simulink model "GTA_PCMFirmware"  (Simulink 7.8)
settings: Solver=FixedStepDiscrete  StartTime=0.0  StopTime=10.0  RelTol=1e-3
PreLoadFcn:
  | try, eval([bdroot '_setup']); catch, eval('model_setup', ''); end
InitFcn:
  | try, eval([bdroot '_setup']); catch, eval('model_setup', ''); end
undefined symbols (not defined in the file): fndFwd, fndNeut, fndRev, FWDlockout, GCM, keySwIgn2, motohawk_build_version, motohawk_trunc_name, motohawk_vardec_path, REVlockout
libraries: MotoHawk_lib x313, simulink x47, GTA_Library x13
(part 1 of 7)
Description:
  | GTA_PCMFirmware
CloseFcn:
  | try, eval([bdroot '_close']); catch, eval('model_close', ''); end
settings Model: MotoHawkBuildVersion=020  MotoHawkBuildStats=struct('TotalFLASH',{0},'TotalEEPROM',{0},'TotalRAM',{0},'AppFLASH',{0},'AppEEPROM',{0},'AppRAM',{0},'HeapRAM',{0},'BuildSuccessCount',{20},'BuildErrorCount',{3})  MotoHawkModelSavedName=GTA_PCMFirmware  MotoHawkModelGUID=31d1e75d-84c7-4dc1-83-eb-d3-41-88-c6-07  MotoHawkModelOpenTime=2012 8 2 11 56 57.463  MotoHawkModelElapsedTime=1635613.383  MotoHawkBuildInfo=struct('model_name',{'GTA_PCMFirmware'},'motohawk_version',{'2011b_sp2.227'},'motohawk_component_version',{'0.0.7'},'matlab_version',{'7.13.0'},'build_version',{'019'},'module_type',{'GCM-0563-048-0802'},'layout_type',{'DEV'},'processor_family',{'PPC'},'processor_type',{'MPC563'},'toolchain_vendor',{'gcc-powerpc-eabi'},'toolchain_version',{'4.6.0'},'component',{0},'archive_file',{'FIRE48.a'},'enable_build',{1},'fptype',{0},'flash_size',{524288},'ee_size',{16384},'ram_size',{32768},'decram_size',{2048},'module_memory_def',{'MPC563_ModMemoryDef_Dev'},'eri_table0_rev',{9},'max_eri_table_size',{65535},'use_debug_vardecs',{1},'use_info_vardecs',{1},'fgnd_base_period_ms',{5},'bgnd_base_period_ms',{50},'root_build_dir',{'D:\Users\pipenberg\Dropbox\WMGTA\Technical\Software\PCM_Firmware\GTA_PCMFirmware'},'build_dir',{'D:\Users\pipenberg\Dropbox\WMGTA\Technical\Software\PCM_Firmware\GTA_PCMFirmware\GTA_PCMFirmware_Build'},'dll_name',{'GTA_PCMFi_019'},'srz_name',{'GTA_PCMFirmware_019'},'fgnd_stack_size',{3072},'fgnd_angle_stack_size',{0},'bgnd_stack_size',{2048},'idle_stack_size',{1024},'irq_stack_size',{1536},'heap_size',{4096},'heap_margin',{409},'install_dll_dir',{'C:\ECUFiles\TDBDLL'},'install_srz_dir',{'C:\ECUFiles\Programs\'},'app_int_stack_size',{1024},'shutdown_stack_size',{1024},'mingw_dir',{'C:\Program Files (x86)\Woodward\DevelopmentTools\Toolchains\GCC\win32-pe\4_4_0\'},'motohawk_dir',{'C:\Program Files (x86)\Woodward\MCS\MotoHawk\2011b_sp2.227'},'toolchain_dir',{'C:\Program Files (x86)\Woodward\DevelopmentTools\Toolchains\GCC\powerpc-eabi\4_6_0'},'matlab_root',{'C:\Program Files\MATLAB\R2011b'},'model_guid',{'31d1e75d-84c7-4dc1-83-eb-d3-41-88-c6-07'},'build_guid',{'afea414d-dbf6-4ed7-b0-f9-6e-db-88-3a-76'},'token_guid',{'71C461C96109B340859695742C634452'})  MotoHawkBuildGUID=afea414d-dbf6-4ed7-b0-f9-6e-db-88-3a-76  Creator=cspenc  LastModifiedBy=pipenberg
settings OptimizationCC: InlineParams=on  InitFltsAndDblsToZero=on  OptimizeModelRefInitCode=on  LifeSpan=1
settings DebuggingCC: SolverPrmCheckMsg=none  InheritedTsInSrcMsg=none  TasksWithSamePriorityMsg=none  FcnCallInpInsideContextMsg=Use local settings  StrictBusMsg=Warning
settings HardwareCC: ProdEndianess=BigEndian  ProdHWDeviceType=Specified
settings RTWCC: SystemTargetFile=motohawk_ert_rtw.tlc  TLCOptions="-aCustomNonFinites=\"motohawk_genrtnonfinite.tlc\""  MakeCommand=motohawk_make_rtw  TemplateMakefile=motohawk_ert_rtw.tmf  Description=MotoHawk(tm) Rapid Prototyping  ProcessScript=motohawk_ert_rtw_make_rtw_hook
settings CodeAppCC: IgnoreCustomStorageClasses=off  MaxIdLength=100  CustomSymbolStrField=$H$N$M
settings STFCustomTargetCC: ModelReferenceCompliant=off  GeneratePreprocessorConditionals=Use local settings  CombineOutputUpdateFcns=on  ERTCustomFileBanners=on  SupportContinuousTime=off  SupportNonInlinedSFcns=off  CPPClassGenCompliant=on  SystemTargetFile=motohawk_ert_rtw.tlc
settings ERTTargetCC: MultiwordLength=2048  ModelReferenceCompliant=off  ParMdlRefBuildCompliant=off  CompOptLevelCompliant=off  ConcurrentExecutionCompliant=off  ERTFirstTimeCompliant=off  ModelStepFunctionPrototypeControlCompliant=off  ERTCustomFileTemplate=example_file_process.tlc  ConvertIfToSwitch=off  SuppressUnreachableDefaultCases=off

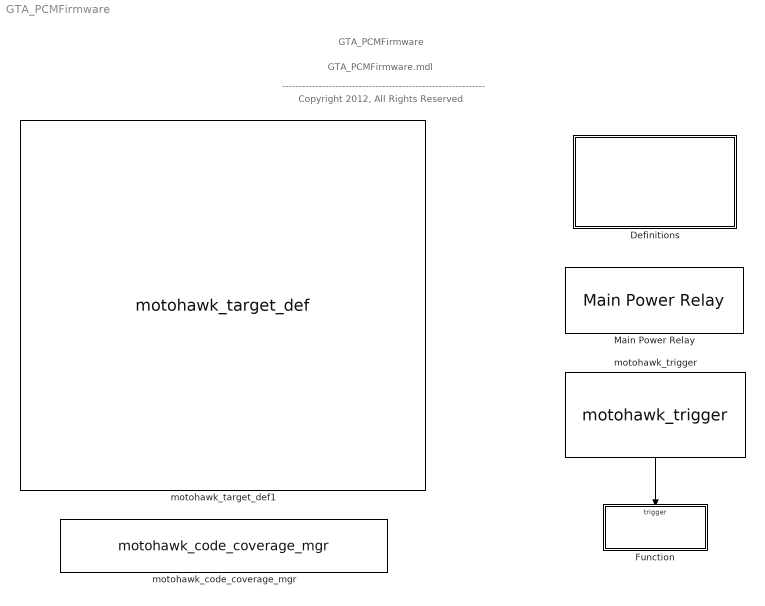
== system GTA_PCMFirmware ==
  note: GTA_PCMFirmware
  note: GTA_PCMFirmware.mdl
  note: -------------------------------------------------------------
  note: Copyright 2012, All Rights Reserved
  Definitions : Subsystem
  Function : Subsystem  TreatAsAtomicUnit=on
      mask init:
      | SampleTime = 0.005;
      | lbl = sprintf('%d ms', SampleTime * 1000);
      settings: RTWSystemCode=Function  RTWFcnNameOpts=Use subsystem name  RTWFileNameOpts=Use function name
      mask Display: disp(lbl);
  Main Power Relay : MotoHawk_lib/Extra Development Blocks/Main Power Relay  on_delay_count=2  off_delay_count=5  ecup_threshold=100  group='System | Main Power Relay'
  motohawk_code_coverage_mgr : MotoHawk_lib/Extra Development Blocks/motohawk_code_coverage_mgr  codegen=Always Generate Code Coverage Code  group='System | Code Coverage'
  motohawk_target_def1 : MotoHawk_lib/motohawk_target_def  Priority=-65535  target=GCM-0563-048-0802  layout=DEV  fptype=single (32 bits)  fgnd_stack_size=3*1024  fgnd_angle_stack_size=0  bgnd_stack_size=2*1024  idle_stack_size=1024  irq_stack_size=1536  app_int_stack_size=1024  shutdown_stack_size=1024  heap_size=4*1024  show_margins=off  fgnd_stack_margin=(3*1024) * 0.1  fgnd_angle_stack_margin=0  bgnd_stack_margin=(2*1024) * 0.1  idle_stack_margin=(1024) * 0.1  irq_stack_margin=(1536) * 0.1  app_int_stack_margin=(1024) * 0.1  shutdown_stack_margin=(1024) * 0.1  heap_margin=(4*1024) * 0.1  comp_name=bdroot  comp_img='KVASER_CAN_USB.jpg'  comp_security=No Encryption  comp_build_pass='mhbuild'  comp_sim_pass='mhsim'  comp_multi=off  show_filenames=off  dll_name=motohawk_trunc_name(bdroot, ['_' motohawk_build_version], 13)  srz_name=motohawk_trunc_name(bdroot, ['_' motohawk_build_version], 50)  build_dir='.'  comp_dir='.'
  motohawk_trigger : MotoHawk_lib/Trigger Blocks/motohawk_trigger  Tag=Trigger  Priority=0  trigger=FGND_RTI_PERIODIC  function_name=Trigger_FGND_RTI_PERIODIC_8744p0012  priority_order=0  inherited=off  run_disabled=off  override_app_monitor=off  target=GCM_0563_048_0802
  wires:
  motohawk_trigger/1 -> Function/Trigger

== system GTA_PCMFirmware/Definitions ==
  CAN Definition : MotoHawk_lib/CAN Blocks/CAN Definition  Priority=-100  nam='CAN_1'  text_resource=CAN1  code_resource=NONE  val_resource=-1  target=GCM-0563-048-0802  bus=-2  btime=500 kbaud  pre=1  prop=0  pseg1=0  pseg2=0  resyn=0  tx_queue_size=16  rx_queue_size=16  use_protocol=on  city_id=hex2dec('B')  access_level=4  mototune_group='System | System Config | Communication Config'
  CAN Definition1 : MotoHawk_lib/CAN Blocks/CAN Definition  Priority=-100  nam='BMS_CAN'  text_resource=CAN2  code_resource=NONE  val_resource=-1  target=GCM-0563-048-0802  bus=-2  btime=500 kbaud  pre=1  prop=0  pseg1=0  pseg2=0  resyn=0  tx_queue_size=16  rx_queue_size=16  use_protocol=on  city_id=hex2dec('B')  access_level=4  mototune_group='System | System Config | Communication Config'
  CAN Definition2 : MotoHawk_lib/CAN Blocks/CAN Definition  Priority=-100  nam='Isolated_CAN'  text_resource=CAN3  code_resource=NONE  val_resource=-1  target=GCM-0563-048-0802  bus=-2  btime=500 kbaud  pre=1  prop=0  pseg1=0  pseg2=0  resyn=0  tx_queue_size=16  rx_queue_size=16  use_protocol=on  city_id=hex2dec('B')  access_level=4  mototune_group='System | System Config | Communication Config'
  Tool Chain Definition : MotoHawk_lib/Build/Tool Chain Definition  nam='MyToolChain'  toolchain=gcc-powerpc-eabi 4.6.0  buildtemplate=GreenHills 3.6  toolchaindir='C:\GHS\ppc421\'  target=GCM-0563-048-0802
  motohawk_trigger_def : MotoHawk_lib/Trigger Blocks/motohawk_trigger_def  fgnd_rti_rate=5000  bgnd_base_multiple=10  read_level=1  write_level=1  mototune_group='System | System Config | Trigger Config'

== system GTA_PCMFirmware/Function ==
  f : TriggerPort  TriggerType=function-call
  1 Inputs and Paramaters : Subsystem
  2 Control Loop : Subsystem
  3 Output and Debug : Subsystem
  motohawk_code_coverage : MotoHawk_lib/Extra Development Blocks/motohawk_code_coverage
  wires:
  1 Inputs and Paramaters/1(Inputs) -> 2 Control Loop/1(Input Bus), 3 Output and Debug/1(InputBus)
  2 Control Loop/1(System Outputs) -> 3 Output and Debug/2(ControlBus)

== system GTA_PCMFirmware/Function/1 Inputs and Paramaters ==
  Analog : Subsystem
  Bus Creator1 : BusCreator  Inputs=5
  CAN : Subsystem
  Digital : Subsystem
  Limits : Subsystem
  SYS Paramaters : Subsystem
  Inputs : Outport
  wires:
  SYS Paramaters/1(SYS Params) -> CAN/1(CAN Params), Limits/1(SysParams), Bus Creator1/1  "SysParams"
  CAN/1(CAN) -> Limits/2(CANin), Bus Creator1/3  "CANin"
  Analog/1(Analog Inputs) -> Bus Creator1/4  "AnalogIn"
  Digital/1(Digital Inputs) -> Bus Creator1/5  "DigitalIn"
  Limits/1(Limits) -> Bus Creator1/2  "Limits"
  Bus Creator1/1 -> Inputs/1

== system GTA_PCMFirmware/Function/2 Control Loop ==
  Input Bus : Inport
  Component Controls : Subsystem
  Mode Control & Ready : Subsystem
  Safety : Subsystem
  System Outputs : Outport
  wires:
  Input Bus/1 -> Safety/1(Input Bus)
  Safety/1(Inputs & Safety) -> Mode Control & Ready/1(Inputs)
  Mode Control & Ready/1(To System Controls) -> Component Controls/1(System Inputs)
  Component Controls/1(System Outputs) -> System Outputs/1

== system GTA_PCMFirmware/Function/3 Output and Debug ==
  InputBus : Inport
  ControlBus : Inport  Port=2
  CAN : Subsystem
  Debug Logic : Subsystem
  Digital : Subsystem
  wires:
  ControlBus/1 -> Digital/1(ControlBus), CAN/3(ControlBus), Debug Logic/2(ControlBus)
  InputBus/1 -> Debug Logic/1(InputBus), CAN/2(InputBus)
  Debug Logic/1(Out1) -> CAN/1(DebugBus)

== system GTA_PCMFirmware/Function/1 Inputs and Paramaters/Analog ==
  Bus Creator : BusCreator  Inputs=3
  Supply Sense : Subsystem
  Throttle Pedal : Subsystem
  Wiper Pot : Subsystem
  Analog Inputs : Outport
  wires:
  Supply Sense/1(Supply) -> Bus Creator/1  "SupplySense"
  Throttle Pedal/1(PedalPerc) -> Bus Creator/2  "ThrottlePedal"
  Wiper Pot/1(WiperPot) -> Bus Creator/3  "WiperPot"
  Bus Creator/1 -> Analog Inputs/1

== system GTA_PCMFirmware/Function/1 Inputs and Paramaters/CAN ==
  CAN Params : Inport
  " Motor Controller" : Subsystem
  BMS : Subsystem
  Bus Creator : BusCreator  Inputs=3
  Charger : Subsystem
  CAN : Outport
  wires:
  CAN Params/1 -> " Motor Controller"/1(CAN Params), BMS/1(CAN Params), Charger/1(CAN Params)
  " Motor Controller"/1(Kinetek) -> Bus Creator/1  "Motor Controller"
  BMS/1(CurrentSensor) -> Bus Creator/2  "BMS"
  Charger/1(Charger) -> Bus Creator/3  "Charger"
  Bus Creator/1 -> CAN/1

== system GTA_PCMFirmware/Function/1 Inputs and Paramaters/Digital ==
  Brake Switch : Subsystem
  Bus Creator : BusCreator  Inputs=7
  Charger : Subsystem
  EStop : Subsystem
  Key Switch : Subsystem
  Rear Defrost Switch : Subsystem
  Shifter : Subsystem
  Wiper Enable : Subsystem
  Digital Inputs : Outport
  wires:
  Brake Switch/1(BrakeSwitch) -> Bus Creator/1  "BrakeSwitch"
  Charger/1(Charger) -> Bus Creator/2  "Charger"
  EStop/1(Estop) -> Bus Creator/3  "EStop"
  Key Switch/1(KeySw) -> Bus Creator/4  "KeySwitch"
  Rear Defrost Switch/1(DefrostSW) -> Bus Creator/5  "RearDefrostSw"
  Wiper Enable/1(WiperSw) -> Bus Creator/7  "WiperSw"
  Shifter/1(Shifter) -> Bus Creator/6  "Shifter"
  Bus Creator/1 -> Digital Inputs/1

== system GTA_PCMFirmware/Function/1 Inputs and Paramaters/Limits ==
  SysParams : Inport
  CANin : Inport  Port=2
  Bus Creator : BusCreator  Inputs=15
  Bus Creator1 : BusCreator  Inputs=1
  Bus Selector : BusSelector  OutputSignals=BMS.csPackSize.PackSize
  Bus Selector1 : BusSelector  OutputSignals=CellTempFaultOffset
  Demux : Demux  Outputs=13
  Li15kWh : Subsystem
  Li23kWh : Subsystem
  Li7kWh : Subsystem
  MinMax : MinMax  Function=max  Inputs=2
  MinMax1 : MinMax  Inputs=2
  Multiport Switch : MultiPortSwitch  Inputs=4  DataPortForDefault=Additional data port  zeroidx=off
  Pb : Subsystem
  Sum : Sum  Inputs=|++
  Sum1 : Sum  Inputs=-+|
  motohawk_probe : MotoHawk_lib/Calibration & Probing Blocks/motohawk_probe  nam='BatterySettings'  show_more=off  name_source=Use Parameter  read_level=1  view_as=Number  enum_struct={'Disabled', 'Enabled'}  vector_style=Wide Row  use_help_units=off  help=''  units=''  use_header_enum=off  row_header_enum={}  col_header_enum={}  use_min_max=off  min_val=-inf  max_val=inf  use_precision=off  precision=''  gain=1  offset=0  exp=1  use_mototune_group=off  mototune_group=motohawk_vardec_path(gcb)
  Limits : Outport
  wires:
  SysParams/1 -> Bus Selector1/1
  CANin/1 -> Bus Selector/1
  Pb/1(PbPack) -> Multiport Switch/5  "PbPack"
  Li7kWh/1(Li7Pack) -> Multiport Switch/2, Multiport Switch/6  "Li7Pack"
  Li15kWh/1(Li15Pack) -> Multiport Switch/3  "Li15Pack"
  Li23kWh/1(Li23Pack) -> Multiport Switch/4  "Li23Pack"
  Bus Selector/1 -> Multiport Switch/1  "<PackSize>"
  Multiport Switch/1 -> Demux/1
  Demux/1 -> Bus Creator/1  "MaxCellVoltage"
  Demux/2 -> Bus Creator/2  "MinCellVoltage"
  Demux/3 -> Bus Creator/3  "CurrentLimit"
  Demux/4 -> Bus Creator/4  "RegenLimit"
  Demux/5 -> Bus Creator/5, MinMax/1  "MaxChargeTemp"
  Demux/6 -> Bus Creator/6, MinMax1/1  "MinChargeTemp"
  Demux/7 -> Bus Creator/7, MinMax/2  "MaxDischargeTemp"
  Demux/8 -> Bus Creator/8, MinMax1/2  "MinDischargeTemp"
  Demux/9 -> Bus Creator/9  "MaxPackVoltage"
  Demux/10 -> Bus Creator/10  "MinPackVoltage"
  Demux/11 -> Bus Creator/11  "MotorCurrentScalar"
  Demux/12 -> Bus Creator/12  "MotorRegenScalar"
  Demux/13 -> Bus Creator/13  "MaxRegenVoltage"
  Bus Creator1/1 -> Limits/1
  Bus Creator/1 -> Bus Creator1/1, motohawk_probe/1  "BattLimits"
  Sum/1 -> Bus Creator/14  "BFmaxCellTemp"
  Sum1/1 -> Bus Creator/15  "BFminCellTemp"
  MinMax/1 -> Sum/1
  Bus Selector1/1 -> Sum/2, Sum1/1  "<CellTempFaultOffset>"
  MinMax1/1 -> Sum1/2

== system GTA_PCMFirmware/Function/1 Inputs and Paramaters/SYS Paramaters ==
  Bus Creator : BusCreator  Inputs=16
  motohawk_calibration : MotoHawk_lib/Calibration & Probing Blocks/motohawk_calibration  nam='CANTimeout'  val=CANTimeout  storage=Calibration  show_more=off  name_source=Use Parameter  data_type=Inherit from 'Default Value'  read_level=1  write_level=1  ovr_cals=on  view_as=Number  enum_struct={'Disabled', 'Enabled'}  vector_style=Wide Row  use_help_units=off  help=''  units=''  use_header_enum=off  row_header_enum={}  col_header_enum={}  use_min_max=off  min_val=-inf  max_val=inf  use_precision=off  precision=''  gain=1  offset=0  exp=1  use_mototune_group=off  mototune_group=motohawk_vardec_path(gcb)
  motohawk_calibration1 : MotoHawk_lib/Calibration & Probing Blocks/motohawk_calibration  nam='MinSOC'  val=MinSOC  storage=Calibration  show_more=off  name_source=Use Parameter  data_type=Inherit from 'Default Value'  read_level=1  write_level=1  ovr_cals=on  view_as=Number  enum_struct={'Disabled', 'Enabled'}  vector_style=Wide Row  use_help_units=off  help=''  units=''  use_header_enum=off  row_header_enum={}  col_header_enum={}  use_min_max=off  min_val=-inf  max_val=inf  use_precision=off  precision=''  gain=1  offset=0  exp=1  use_mototune_group=off  mototune_group=motohawk_vardec_path(gcb)
  motohawk_calibration10 : MotoHawk_lib/Calibration & Probing Blocks/motohawk_calibration  nam='CellVoltageTaper'  val=CellVoltageTaper  storage=Calibration  show_more=off  name_source=Use Parameter  data_type=Inherit from 'Default Value'  read_level=1  write_level=1  ovr_cals=on  view_as=Number  enum_struct={'Disabled', 'Enabled'}  vector_style=Wide Row  use_help_units=off  help=''  units=''  use_header_enum=off  row_header_enum={}  col_header_enum={}  use_min_max=off  min_val=-inf  max_val=inf  use_precision=off  precision=''  gain=1  offset=0  exp=1  use_mototune_group=off  mototune_group=motohawk_vardec_path(gcb)
  motohawk_calibration11 : MotoHawk_lib/Calibration & Probing Blocks/motohawk_calibration  nam='CellVoltDB'  val=CellVoltDB  storage=Calibration  show_more=off  name_source=Use Parameter  data_type=Inherit from 'Default Value'  read_level=1  write_level=1  ovr_cals=on  view_as=Number  enum_struct={'Disabled', 'Enabled'}  vector_style=Wide Row  use_help_units=off  help=''  units=''  use_header_enum=off  row_header_enum={}  col_header_enum={}  use_min_max=off  min_val=-inf  max_val=inf  use_precision=off  precision=''  gain=1  offset=0  exp=1  use_mototune_group=off  mototune_group=motohawk_vardec_path(gcb)
  motohawk_calibration12 : MotoHawk_lib/Calibration & Probing Blocks/motohawk_calibration  nam='CellTempFaultOffset'  val=CellTempFaultOffset  storage=Calibration  show_more=off  name_source=Use Parameter  data_type=Inherit from 'Default Value'  read_level=1  write_level=1  ovr_cals=on  view_as=Number  enum_struct={'Disabled', 'Enabled'}  vector_style=Wide Row  use_help_units=off  help=''  units=''  use_header_enum=off  row_header_enum={}  col_header_enum={}  use_min_max=off  min_val=-inf  max_val=inf  use_precision=off  precision=''  gain=1  offset=0  exp=1  use_mototune_group=off  mototune_group=motohawk_vardec_path(gcb)
  motohawk_calibration13 : MotoHawk_lib/Calibration & Probing Blocks/motohawk_calibration  nam='maxMotorRPM'  val=maxMotorRPM  storage=Calibration  show_more=off  name_source=Use Parameter  data_type=Inherit from 'Default Value'  read_level=1  write_level=1  ovr_cals=on  view_as=Number  enum_struct={'Disabled', 'Enabled'}  vector_style=Wide Row  use_help_units=off  help=''  units=''  use_header_enum=off  row_header_enum={}  col_header_enum={}  use_min_max=off  min_val=-inf  max_val=inf  use_precision=off  precision=''  gain=1  offset=0  exp=1  use_mototune_group=off  mototune_group=motohawk_vardec_path(gcb)
  motohawk_calibration14 : MotoHawk_lib/Calibration & Probing Blocks/motohawk_calibration  nam='invOverTemp'  val=invOverTemp  storage=Calibration  show_more=off  name_source=Use Parameter  data_type=Inherit from 'Default Value'  read_level=1  write_level=1  ovr_cals=on  view_as=Number  enum_struct={'Disabled', 'Enabled'}  vector_style=Wide Row  use_help_units=off  help=''  units=''  use_header_enum=off  row_header_enum={}  col_header_enum={}  use_min_max=off  min_val=-inf  max_val=inf  use_precision=off  precision=''  gain=1  offset=0  exp=1  use_mototune_group=off  mototune_group=motohawk_vardec_path(gcb)
  motohawk_calibration15 : MotoHawk_lib/Calibration & Probing Blocks/motohawk_calibration  nam='motorOverTemp'  val=motorOverTemp  storage=Calibration  show_more=off  name_source=Use Parameter  data_type=Inherit from 'Default Value'  read_level=1  write_level=1  ovr_cals=on  view_as=Number  enum_struct={'Disabled', 'Enabled'}  vector_style=Wide Row  use_help_units=off  help=''  units=''  use_header_enum=off  row_header_enum={}  col_header_enum={}  use_min_max=off  min_val=-inf  max_val=inf  use_precision=off  precision=''  gain=1  offset=0  exp=1  use_mototune_group=off  mototune_group=motohawk_vardec_path(gcb)
  motohawk_calibration2 : MotoHawk_lib/Calibration & Probing Blocks/motohawk_calibration  nam='CellTempTaper'  val=CellTempTaper  storage=Calibration  show_more=off  name_source=Use Parameter  data_type=Inherit from 'Default Value'  read_level=1  write_level=1  ovr_cals=on  view_as=Number  enum_struct={'Disabled', 'Enabled'}  vector_style=Wide Row  use_help_units=off  help=''  units=''  use_header_enum=off  row_header_enum={}  col_header_enum={}  use_min_max=off  min_val=-inf  max_val=inf  use_precision=off  precision=''  gain=1  offset=0  exp=1  use_mototune_group=off  mototune_group=motohawk_vardec_path(gcb)
  motohawk_calibration3 : MotoHawk_lib/Calibration & Probing Blocks/motohawk_calibration  nam='PackVoltageTaper'  val=PackVoltageTaper  storage=Calibration  show_more=off  name_source=Use Parameter  data_type=Inherit from 'Default Value'  read_level=1  write_level=1  ovr_cals=on  view_as=Number  enum_struct={'Disabled', 'Enabled'}  vector_style=Wide Row  use_help_units=off  help=''  units=''  use_header_enum=off  row_header_enum={}  col_header_enum={}  use_min_max=off  min_val=-inf  max_val=inf  use_precision=off  precision=''  gain=1  offset=0  exp=1  use_mototune_group=off  mototune_group=motohawk_vardec_path(gcb)
  motohawk_calibration4 : MotoHawk_lib/Calibration & Probing Blocks/motohawk_calibration  nam='PackCurrentTaper'  val=PackCurrentTaper  storage=Calibration  show_more=off  name_source=Use Parameter  data_type=Inherit from 'Default Value'  read_level=1  write_level=1  ovr_cals=on  view_as=Number  enum_struct={'Disabled', 'Enabled'}  vector_style=Wide Row  use_help_units=off  help=''  units=''  use_header_enum=off  row_header_enum={}  col_header_enum={}  use_min_max=off  min_val=-inf  max_val=inf  use_precision=off  precision=''  gain=1  offset=0  exp=1  use_mototune_group=off  mototune_group=motohawk_vardec_path(gcb)
  motohawk_calibration5 : MotoHawk_lib/Calibration & Probing Blocks/motohawk_calibration  nam='LowSOCcurrLimit'  val=LowSOCcurrLimit  storage=Calibration  show_more=off  name_source=Use Parameter  data_type=Inherit from 'Default Value'  read_level=1  write_level=1  ovr_cals=on  view_as=Number  enum_struct={'Disabled', 'Enabled'}  vector_style=Wide Row  use_help_units=off  help=''  units=''  use_header_enum=off  row_header_enum={}  col_header_enum={}  use_min_max=off  min_val=-inf  max_val=inf  use_precision=off  precision=''  gain=1  offset=0  exp=1  use_mototune_group=off  mototune_group=motohawk_vardec_path(gcb)
  motohawk_calibration6 : MotoHawk_lib/Calibration & Probing Blocks/motohawk_calibration  nam='HighSpeedLimit'  val=HighSpeedLimit  storage=Calibration  show_more=off  name_source=Use Parameter  data_type=Inherit from 'Default Value'  read_level=1  write_level=1  ovr_cals=on  view_as=Number  enum_struct={'Disabled', 'Enabled'}  vector_style=Wide Row  use_help_units=off  help=''  units=''  use_header_enum=off  row_header_enum={}  col_header_enum={}  use_min_max=off  min_val=-inf  max_val=inf  use_precision=off  precision=''  gain=1  offset=0  exp=1  use_mototune_group=off  mototune_group=motohawk_vardec_path(gcb)
  motohawk_calibration7 : MotoHawk_lib/Calibration & Probing Blocks/motohawk_calibration  nam='LowSpeedLimit'  val=LowSpeedLimit  storage=Calibration  show_more=off  name_source=Use Parameter  data_type=Inherit from 'Default Value'  read_level=1  write_level=1  ovr_cals=on  view_as=Number  enum_struct={'Disabled', 'Enabled'}  vector_style=Wide Row  use_help_units=off  help=''  units=''  use_header_enum=off  row_header_enum={}  col_header_enum={}  use_min_max=off  min_val=-inf  max_val=inf  use_precision=off  precision=''  gain=1  offset=0  exp=1  use_mototune_group=off  mototune_group=motohawk_vardec_path(gcb)
  motohawk_calibration8 : MotoHawk_lib/Calibration & Probing Blocks/motohawk_calibration  nam='RevSpeedLimit'  val=RevSpeedLimit  storage=Calibration  show_more=off  name_source=Use Parameter  data_type=Inherit from 'Default Value'  read_level=1  write_level=1  ovr_cals=on  view_as=Number  enum_struct={'Disabled', 'Enabled'}  vector_style=Wide Row  use_help_units=off  help=''  units=''  use_header_enum=off  row_header_enum={}  col_header_enum={}  use_min_max=off  min_val=-inf  max_val=inf  use_precision=off  precision=''  gain=1  offset=0  exp=1  use_mototune_group=off  mototune_group=motohawk_vardec_path(gcb)
  motohawk_calibration9 : MotoHawk_lib/Calibration & Probing Blocks/motohawk_calibration  nam='SpeedTaper'  val=SpeedTaper  storage=Calibration  show_more=off  name_source=Use Parameter  data_type=Inherit from 'Default Value'  read_level=1  write_level=1  ovr_cals=on  view_as=Number  enum_struct={'Disabled', 'Enabled'}  vector_style=Wide Row  use_help_units=off  help=''  units=''  use_header_enum=off  row_header_enum={}  col_header_enum={}  use_min_max=off  min_val=-inf  max_val=inf  use_precision=off  precision=''  gain=1  offset=0  exp=1  use_mototune_group=off  mototune_group=motohawk_vardec_path(gcb)
  SYS Params : Outport
  wires:
  motohawk_calibration/1 -> Bus Creator/1  "CANTimeout"
  Bus Creator/1 -> SYS Params/1
  motohawk_calibration1/1 -> Bus Creator/2  "MinSOC"
  motohawk_calibration3/1 -> Bus Creator/5  "PackVoltageTaper"
  motohawk_calibration2/1 -> Bus Creator/3  "CellTempTaper"
  motohawk_calibration4/1 -> Bus Creator/6  "PackCurrentTaper"
  motohawk_calibration5/1 -> Bus Creator/7  "LowSOCcurrLimit"
  motohawk_calibration6/1 -> Bus Creator/8  "HighSpeedLimit"
  motohawk_calibration7/1 -> Bus Creator/9  "LowSpeedLimit"
  motohawk_calibration8/1 -> Bus Creator/10  "RevSpeedLimit"
  motohawk_calibration9/1 -> Bus Creator/11  "SpeedTaper"
  motohawk_calibration10/1 -> Bus Creator/12  "CellVoltageTaper"
  motohawk_calibration11/1 -> Bus Creator/13  "CellVoltDB"
  motohawk_calibration12/1 -> Bus Creator/4  "CellTempFaultOffset"
  motohawk_calibration13/1 -> Bus Creator/14  "maxMotorRPM"
  motohawk_calibration14/1 -> Bus Creator/15  "invOverTemp"
  motohawk_calibration15/1 -> Bus Creator/16  "motorOverTemp"

== system GTA_PCMFirmware/Function/2 Control Loop/Component Controls ==
  System Inputs : Inport
  Body Control : Subsystem
  Bus Creator : BusCreator  Inputs=5
  Charger Control : Subsystem
  Display Control : Subsystem
  Motor Control : Subsystem
  System Outputs : Outport
  wires:
  System Inputs/1 -> Display Control/1(SYSin), Charger Control/1(SYSin), Body Control/1(SYSin), Motor Control/1(SYSin), Bus Creator/1  "SYSin"
  Display Control/1(Out) -> Bus Creator/2  "Display"
  Motor Control/1(Out) -> Bus Creator/5, Body Control/2(MotorControl), Display Control/2(MotorControl)  "MotorControl"
  Body Control/1(Out) -> Bus Creator/4  "BodyControl"
  Charger Control/1(Out) -> Bus Creator/3  "Charger"
  Bus Creator/1 -> System Outputs/1

== system GTA_PCMFirmware/Function/2 Control Loop/Mode Control & Ready ==
  Inputs : Inport
  Bus Creator : BusCreator  Inputs=3
  Mode Control : Subsystem
  Ready : Subsystem
  To System Controls : Outport
  wires:
  Inputs/1 -> Ready/1(Inputs), Mode Control/2(Bus In), Bus Creator/1  "BUS"
  Ready/1(Ready) -> Mode Control/1(Ready), Bus Creator/2  "ReadyState"
  Mode Control/1(ModeControlOut) -> Bus Creator/3  "ModeControl"
  Bus Creator/1 -> To System Controls/1

== system GTA_PCMFirmware/Function/2 Control Loop/Safety ==
  Input Bus : Inport
  Bus Creator : BusCreator
  Bus Creator1 : BusCreator  Inputs=2
  Bus Creator2 : BusCreator  Inputs=1
  Current Limit : Subsystem
  Faults : Subsystem
  Voltage Level : Subsystem
  Inputs & Safety : Outport
  wires:
  Input Bus/1 -> Bus Creator/1, Bus Creator1/1, Voltage Level/1(Input Bus), Bus Creator2/1  "Input Bus"
  Voltage Level/1(Out1) -> Bus Creator/4, Bus Creator1/2  "Voltage level"
  Bus Creator/1 -> Inputs & Safety/1
  Bus Creator1/1 -> Current Limit/1(Input Bus)
  Current Limit/1(CurrentLimits) -> Bus Creator/3  "Current Limit"
  Faults/1(Out1) -> Bus Creator/2  "Faults"
  Bus Creator2/1 -> Faults/1(Input Bus)

== system GTA_PCMFirmware/Function/3 Output and Debug/CAN ==
  DebugBus : Inport
  InputBus : Inport  Port=2
  ControlBus : Inport  Port=3
  Charger : Subsystem
  Current Sensor : Subsystem
  Debug : Subsystem
  Ground : Ground
  Ground1 : Ground
  Instrument Cluster : Subsystem
  MotorController : Subsystem
  wires:
  ControlBus/1 -> MotorController/2(ControlBus), Instrument Cluster/2(ControlBus)
  InputBus/1 -> MotorController/1(InputBus), Instrument Cluster/1(InputBus)
  DebugBus/1 -> Debug/1(Debug In)
  Ground/1 -> Charger/1(null)
  Ground1/1 -> Current Sensor/1(null)

== system GTA_PCMFirmware/Function/3 Output and Debug/Debug Logic ==
  InputBus : Inport
  ControlBus : Inport  Port=2
  Bus Creator : BusCreator  Inputs=3
  Bus Creator1 : BusCreator
  IGN1 Logic : Subsystem
  InverterOT : Subsystem
  MotorOT : Subsystem
  SOCok : Subsystem
  Out1 : Outport
  wires:
  InputBus/1 -> Bus Creator/1, IGN1 Logic/1(InputBus), SOCok/1(InputBus), InverterOT/1(InputBus), MotorOT/1(InputBus)  "InputBus"
  ControlBus/1 -> Bus Creator/2  "ControlBus"
  Bus Creator/1 -> Out1/1
  Bus Creator1/1 -> Bus Creator/3  "DebugBus"
  IGN1 Logic/1(Ign1) -> Bus Creator1/1  "IGN1"
  SOCok/1(SOCok) -> Bus Creator1/2  "SOCok"
  InverterOT/1(InverterOT) -> Bus Creator1/3  "DBGinverterOT"
  MotorOT/1(MotorOT) -> Bus Creator1/4  "DBGmotorOT"

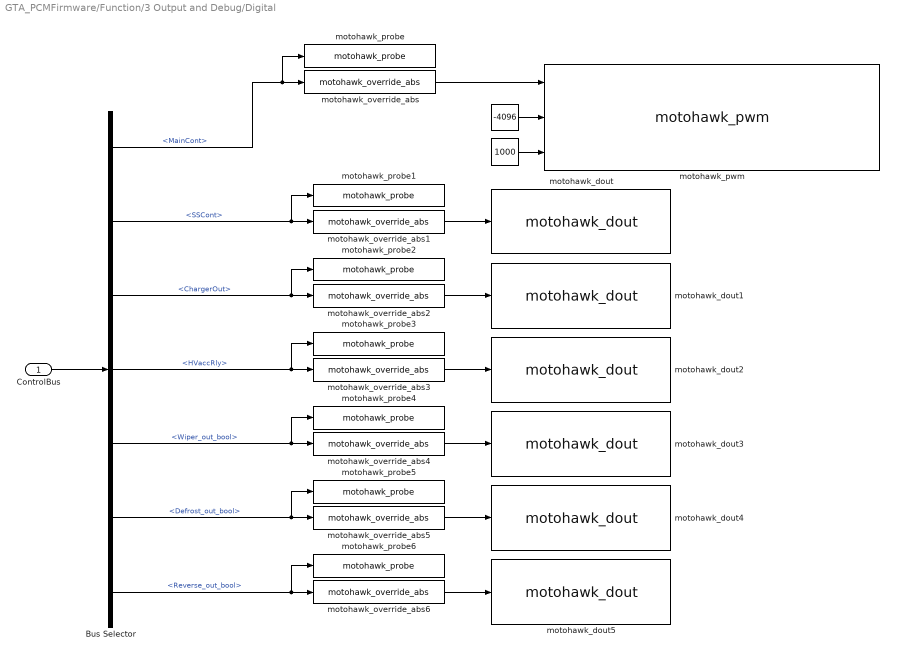
== system GTA_PCMFirmware/Function/3 Output and Debug/Digital ==
  ControlBus : Inport
  " " : Constant  Value=-4096  OutDataTypeStr=int16
  "   " : Constant  Value=1000  OutDataTypeStr=uint32
  Bus Selector : BusSelector  OutputSignals=SYSin.ModeControl.MainCont,SYSin.ModeControl.SSCont,Charger.ChargerOut,SYSin.ModeControl.HVaccRly,BodyControl.Wiper.Wiper_out_bool,BodyControl.Defrost.Defrost_out_bool,BodyControl.ReverseLight.Reverse_out_bool
  motohawk_dout : MotoHawk_lib/Digital I//O Blocks/motohawk_dout  resource_name='prechargeCont'  text_resource=HSD1  target=GCM-0563-048-0802  use_diag=off  use_vardec=off  nam='DOUT'  read_level=1  write_level=1  group='System | I/O Pins | Outputs Config'
  motohawk_dout1 : MotoHawk_lib/Digital I//O Blocks/motohawk_dout  resource_name='Charger_Enable'  text_resource=LSD3  target=GCM-0563-048-0802  use_diag=off  use_vardec=off  nam='DOUT'  read_level=1  write_level=1  group='System | I/O Pins | Outputs Config'
  motohawk_dout2 : MotoHawk_lib/Digital I//O Blocks/motohawk_dout  resource_name='HVaccRly'  text_resource=LSD4  target=GCM-0563-048-0802  use_diag=off  use_vardec=off  nam='DOUT'  read_level=1  write_level=1  group='System | I/O Pins | Outputs Config'
  motohawk_dout3 : MotoHawk_lib/Digital I//O Blocks/motohawk_dout  resource_name='WiperOut'  text_resource=LSD1  target=GCM-0563-048-0802  use_diag=off  use_vardec=off  nam='DOUT'  read_level=1  write_level=1  group='System | I/O Pins | Outputs Config'
  motohawk_dout4 : MotoHawk_lib/Digital I//O Blocks/motohawk_dout  resource_name='DefrostOut'  text_resource=LSD5  target=GCM-0563-048-0802  use_diag=off  use_vardec=off  nam='DOUT'  read_level=1  write_level=1  group='System | I/O Pins | Outputs Config'
  motohawk_dout5 : MotoHawk_lib/Digital I//O Blocks/motohawk_dout  resource_name='ReverseOut'  text_resource=LSD7  target=GCM-0563-048-0802  use_diag=off  use_vardec=off  nam='DOUT'  read_level=1  write_level=1  group='System | I/O Pins | Outputs Config'
  motohawk_override_abs : MotoHawk_lib/Calibration & Probing Blocks/motohawk_override_abs  parent_name='MainContOR'  parent_val=0  show_more=off  name_source=Use Parameter  parent_read_level=1  parent_override_level=1  view_as=Number  enum_struct={'Disabled', 'Enabled'}  use_help_units=off  parent_help=''  parent_units=''  use_min_max=off  parent_min=-inf  parent_max=inf  use_precision=off  parent_precision=''  parent_gain=1  parent_offset=0  parent_exp=1  use_mototune_group=off  parent_group=motohawk_vardec_path(gcb)
  motohawk_override_abs1 : MotoHawk_lib/Calibration & Probing Blocks/motohawk_override_abs  parent_name='prechargeContOR'  parent_val=0  show_more=off  name_source=Use Parameter  parent_read_level=1  parent_override_level=1  view_as=Number  enum_struct={'Disabled', 'Enabled'}  use_help_units=off  parent_help=''  parent_units=''  use_min_max=off  parent_min=-inf  parent_max=inf  use_precision=off  parent_precision=''  parent_gain=1  parent_offset=0  parent_exp=1  use_mototune_group=off  parent_group=motohawk_vardec_path(gcb)
  motohawk_override_abs2 : MotoHawk_lib/Calibration & Probing Blocks/motohawk_override_abs  parent_name='Charger_EnableOR'  parent_val=0  show_more=off  name_source=Use Parameter  parent_read_level=1  parent_override_level=1  view_as=Number  enum_struct={'Disabled', 'Enabled'}  use_help_units=off  parent_help=''  parent_units=''  use_min_max=off  parent_min=-inf  parent_max=inf  use_precision=off  parent_precision=''  parent_gain=1  parent_offset=0  parent_exp=1  use_mototune_group=off  parent_group=motohawk_vardec_path(gcb)
  motohawk_override_abs3 : MotoHawk_lib/Calibration & Probing Blocks/motohawk_override_abs  parent_name='HVaccRlyOR'  parent_val=0  show_more=off  name_source=Use Parameter  parent_read_level=1  parent_override_level=1  view_as=Number  enum_struct={'Disabled', 'Enabled'}  use_help_units=off  parent_help=''  parent_units=''  use_min_max=off  parent_min=-inf  parent_max=inf  use_precision=off  parent_precision=''  parent_gain=1  parent_offset=0  parent_exp=1  use_mototune_group=off  parent_group=motohawk_vardec_path(gcb)
  motohawk_override_abs4 : MotoHawk_lib/Calibration & Probing Blocks/motohawk_override_abs  parent_name='WiperOutOR'  parent_val=0  show_more=off  name_source=Use Parameter  parent_read_level=1  parent_override_level=1  view_as=Number  enum_struct={'Disabled', 'Enabled'}  use_help_units=off  parent_help=''  parent_units=''  use_min_max=off  parent_min=-inf  parent_max=inf  use_precision=off  parent_precision=''  parent_gain=1  parent_offset=0  parent_exp=1  use_mototune_group=off  parent_group=motohawk_vardec_path(gcb)
  motohawk_override_abs5 : MotoHawk_lib/Calibration & Probing Blocks/motohawk_override_abs  parent_name='DefrostOutOR'  parent_val=0  show_more=off  name_source=Use Parameter  parent_read_level=1  parent_override_level=1  view_as=Number  enum_struct={'Disabled', 'Enabled'}  use_help_units=off  parent_help=''  parent_units=''  use_min_max=off  parent_min=-inf  parent_max=inf  use_precision=off  parent_precision=''  parent_gain=1  parent_offset=0  parent_exp=1  use_mototune_group=off  parent_group=motohawk_vardec_path(gcb)
  motohawk_override_abs6 : MotoHawk_lib/Calibration & Probing Blocks/motohawk_override_abs  parent_name='ReverseOutOR'  parent_val=0  show_more=off  name_source=Use Parameter  parent_read_level=1  parent_override_level=1  view_as=Number  enum_struct={'Disabled', 'Enabled'}  use_help_units=off  parent_help=''  parent_units=''  use_min_max=off  parent_min=-inf  parent_max=inf  use_precision=off  parent_precision=''  parent_gain=1  parent_offset=0  parent_exp=1  use_mototune_group=off  parent_group=motohawk_vardec_path(gcb)
  motohawk_probe : MotoHawk_lib/Calibration & Probing Blocks/motohawk_probe  nam='MainContProbe'  show_more=off  name_source=Use Parameter  read_level=1  view_as=Number  enum_struct={'Disabled', 'Enabled'}  vector_style=Wide Row  use_help_units=off  help=''  units=''  use_header_enum=off  row_header_enum={}  col_header_enum={}  use_min_max=off  min_val=-inf  max_val=inf  use_precision=off  precision=''  gain=1  offset=0  exp=1  use_mototune_group=off  mototune_group=motohawk_vardec_path(gcb)
  motohawk_probe1 : MotoHawk_lib/Calibration & Probing Blocks/motohawk_probe  nam='prechargeContProbe'  show_more=off  name_source=Use Parameter  read_level=1  view_as=Number  enum_struct={'Disabled', 'Enabled'}  vector_style=Wide Row  use_help_units=off  help=''  units=''  use_header_enum=off  row_header_enum={}  col_header_enum={}  use_min_max=off  min_val=-inf  max_val=inf  use_precision=off  precision=''  gain=1  offset=0  exp=1  use_mototune_group=off  mototune_group=motohawk_vardec_path(gcb)
  motohawk_probe2 : MotoHawk_lib/Calibration & Probing Blocks/motohawk_probe  nam='Charger_EnableProbe'  show_more=off  name_source=Use Parameter  read_level=1  view_as=Number  enum_struct={'Disabled', 'Enabled'}  vector_style=Wide Row  use_help_units=off  help=''  units=''  use_header_enum=off  row_header_enum={}  col_header_enum={}  use_min_max=off  min_val=-inf  max_val=inf  use_precision=off  precision=''  gain=1  offset=0  exp=1  use_mototune_group=off  mototune_group=motohawk_vardec_path(gcb)
  motohawk_probe3 : MotoHawk_lib/Calibration & Probing Blocks/motohawk_probe  nam='HVaccRlyProbe'  show_more=off  name_source=Use Parameter  read_level=1  view_as=Number  enum_struct={'Disabled', 'Enabled'}  vector_style=Wide Row  use_help_units=off  help=''  units=''  use_header_enum=off  row_header_enum={}  col_header_enum={}  use_min_max=off  min_val=-inf  max_val=inf  use_precision=off  precision=''  gain=1  offset=0  exp=1  use_mototune_group=off  mototune_group=motohawk_vardec_path(gcb)
  motohawk_probe4 : MotoHawk_lib/Calibration & Probing Blocks/motohawk_probe  nam='WiperOutProbe'  show_more=off  name_source=Use Parameter  read_level=1  view_as=Number  enum_struct={'Disabled', 'Enabled'}  vector_style=Wide Row  use_help_units=off  help=''  units=''  use_header_enum=off  row_header_enum={}  col_header_enum={}  use_min_max=off  min_val=-inf  max_val=inf  use_precision=off  precision=''  gain=1  offset=0  exp=1  use_mototune_group=off  mototune_group=motohawk_vardec_path(gcb)
  motohawk_probe5 : MotoHawk_lib/Calibration & Probing Blocks/motohawk_probe  nam='DefrostOutProbe'  show_more=off  name_source=Use Parameter  read_level=1  view_as=Number  enum_struct={'Disabled', 'Enabled'}  vector_style=Wide Row  use_help_units=off  help=''  units=''  use_header_enum=off  row_header_enum={}  col_header_enum={}  use_min_max=off  min_val=-inf  max_val=inf  use_precision=off  precision=''  gain=1  offset=0  exp=1  use_mototune_group=off  mototune_group=motohawk_vardec_path(gcb)
  motohawk_probe6 : MotoHawk_lib/Calibration & Probing Blocks/motohawk_probe  nam='ReverseOutProbe'  show_more=off  name_source=Use Parameter  read_level=1  view_as=Number  enum_struct={'Disabled', 'Enabled'}  vector_style=Wide Row  use_help_units=off  help=''  units=''  use_header_enum=off  row_header_enum={}  col_header_enum={}  use_min_max=off  min_val=-inf  max_val=inf  use_precision=off  precision=''  gain=1  offset=0  exp=1  use_mototune_group=off  mototune_group=motohawk_vardec_path(gcb)
  motohawk_pwm : MotoHawk_lib/Analog I//O Blocks/motohawk_pwm  res_name='MainContactor'  text_resource=H1  target=GCM-0563-048-0802  freq_mode=-1  min_freq=2  use_max_freq=on  max_freq=1000  use_enable=on  use_brake=off  output_current=off  output_fault_status=off  use_child=off  use_vardec=off  nam='PWMOutput'  read_level=1  write_level=1  group='System | I/O Pins | Outputs Config'
  wires:
  " "/1 -> motohawk_pwm/2
  "   "/1 -> motohawk_pwm/3
  motohawk_override_abs1/1 -> motohawk_dout/1
  motohawk_override_abs2/1 -> motohawk_dout1/1
  motohawk_override_abs3/1 -> motohawk_dout2/1
  motohawk_override_abs4/1 -> motohawk_dout3/1
  motohawk_override_abs5/1 -> motohawk_dout4/1
  motohawk_override_abs6/1 -> motohawk_dout5/1
  Bus Selector/2 -> motohawk_override_abs1/1, motohawk_probe1/1  "<SSCont>"
  Bus Selector/5 -> motohawk_override_abs4/1, motohawk_probe4/1  "<Wiper_out_bool>"
  Bus Selector/7 -> motohawk_override_abs6/1, motohawk_probe6/1  "<Reverse_out_bool>"
  motohawk_override_abs/1 -> motohawk_pwm/1
  ControlBus/1 -> Bus Selector/1
  Bus Selector/4 -> motohawk_override_abs3/1, motohawk_probe3/1  "<HVaccRly>"
  Bus Selector/3 -> motohawk_override_abs2/1, motohawk_probe2/1  "<ChargerOut>"
  Bus Selector/1 -> motohawk_override_abs/1, motohawk_probe/1  "<MainCont>"
  Bus Selector/6 -> motohawk_override_abs5/1, motohawk_probe5/1  "<Defrost_out_bool>"

== system GTA_PCMFirmware/Function/1 Inputs and Paramaters/Analog/Supply Sense ==
  Bus Creator : BusCreator  Inputs=1
  Gain : Gain  Gain=5/1023  OutDataTypeStr=single
  Gain1 : Gain  Gain=1/.118  OutDataTypeStr=single
  motohawk_ain_read : MotoHawk_lib/Analog I//O Blocks/motohawk_ain_read  nam='ECUP'  typ=uint16
  motohawk_probe : MotoHawk_lib/Calibration & Probing Blocks/motohawk_probe  nam='V12Ref'  show_more=off  name_source=Use Parameter  read_level=1  view_as=Number  enum_struct={'Disabled', 'Enabled'}  vector_style=Wide Row  use_help_units=off  help=''  units=''  use_header_enum=off  row_header_enum={}  col_header_enum={}  use_min_max=off  min_val=-inf  max_val=inf  use_precision=off  precision=''  gain=1  offset=0  exp=1  use_mototune_group=off  mototune_group=motohawk_vardec_path(gcb)
  Supply : Outport
  wires:
  motohawk_ain_read/1 -> Gain/1
  Gain/1 -> Gain1/1
  Gain1/1 -> Bus Creator/1, motohawk_probe/1  "12VSense"
  Bus Creator/1 -> Supply/1

== system GTA_PCMFirmware/Function/1 Inputs and Paramaters/Analog/Throttle Pedal ==
  Bus Creator : BusCreator  Inputs=2
  Demux : Demux  Outputs=3
  FilterAndNormalize : Subsystem
  Mux : Mux  Inputs=3
  ThrottlePedal : Subsystem
  motohawk_ain : MotoHawk_lib/Analog I//O Blocks/motohawk_ain  res_name='PedalInput1'  text_resource=AN8M  code_resource=NONE  val_resource=-1  target=GCM-0563-048-0802  resource_enum_str=(None)=-1,LSD1=25,LSD2=26,ECUP=53,DRVP=54,XDRP=55,AN1M=56,AN2M=57,AN3M=58,AN4M=59,AN5M=60,AN6M=61,AN7M=62,AN8M=63,AN9M=64,AN10M=65,AN11M=66,AN12M=67,AN13M=68,AN14M=69,AN15M=70,AN16M=71,ESTOP=97,PWMADC=142  altref=5V Reference  typ=uint16  num_adc_bits=12  use_stat=off  use_vardec=off  nam='RTD1_MW'  read_level=1  write_level=1  group='System | I/O Pins | Inputs Config'
  motohawk_ain1 : MotoHawk_lib/Analog I//O Blocks/motohawk_ain  res_name='PedalSupply'  text_resource=XDRP  code_resource=NONE  val_resource=-1  target=GCM-0563-048-0802  resource_enum_str=(None)=-1,LSD1=25,LSD2=26,ECUP=53,DRVP=54,XDRP=55,AN1M=56,AN2M=57,AN3M=58,AN4M=59,AN5M=60,AN6M=61,AN7M=62,AN8M=63,AN9M=64,AN10M=65,AN11M=66,AN12M=67,AN13M=68,AN14M=69,AN15M=70,AN16M=71,ESTOP=97,PWMADC=142  altref=5V Reference  typ=uint16  num_adc_bits=12  use_stat=off  use_vardec=off  nam='RTD1_MW'  read_level=1  write_level=1  group='System | I/O Pins | Inputs Config'
  motohawk_ain2 : MotoHawk_lib/Analog I//O Blocks/motohawk_ain  res_name='PedalInput2'  text_resource=AN9M  code_resource=NONE  val_resource=-1  target=GCM-0563-048-0802  resource_enum_str=(None)=-1,LSD1=25,LSD2=26,ECUP=53,DRVP=54,XDRP=55,AN1M=56,AN2M=57,AN3M=58,AN4M=59,AN5M=60,AN6M=61,AN7M=62,AN8M=63,AN9M=64,AN10M=65,AN11M=66,AN12M=67,AN13M=68,AN14M=69,AN15M=70,AN16M=71,ESTOP=97,PWMADC=142  altref=5V Reference  typ=uint16  num_adc_bits=12  use_stat=off  use_vardec=off  nam='RTD1_MW'  read_level=1  write_level=1  group='System | I/O Pins | Inputs Config'
  PedalPerc : Outport
  wires:
  motohawk_ain/1 -> Mux/1
  motohawk_ain1/1 -> Mux/2
  motohawk_ain2/1 -> Mux/3
  Mux/1 -> FilterAndNormalize/1(In1)
  FilterAndNormalize/1(Out1) -> Demux/1
  Demux/1 -> ThrottlePedal/1(Pedal1)  "Peadl1Filt"
  Demux/3 -> ThrottlePedal/3(Pedal2)  "Pedal2Filt"
  Demux/2 -> ThrottlePedal/2(Supply)  "PedalSupply"
  ThrottlePedal/1(ThrottlePerc) -> Bus Creator/1  "PedalPerc"
  ThrottlePedal/2(NoErr) -> Bus Creator/2  "dbgAPPok"
  Bus Creator/1 -> PedalPerc/1

== system GTA_PCMFirmware/Function/1 Inputs and Paramaters/Analog/Wiper Pot ==
  Bus Creator : BusCreator  Inputs=1
  Data Type Conversion : DataTypeConversion  OutDataTypeStr=single
  Data Type Conversion1 : DataTypeConversion  OutDataTypeStr=single
  Divide : Product  Inputs=*/
  Gain : Gain  Gain=100
  Saturation : Saturate  UpperLimit=100  LowerLimit=0
  Wiper Lookup Table : Lookup_n-D  NumberOfTableDimensions=1  BreakpointsForDimension1=[0 50 78 96 109 119 122]  Table=[0 17 34 50 67 84 100]  RndMeth=Simplest  InputSameDT=on
  motohawk_ain : MotoHawk_lib/Analog I//O Blocks/motohawk_ain  res_name='WiperPot'  text_resource=AN10M  code_resource=NONE  val_resource=-1  target=GCM-0563-048-0802  resource_enum_str=(None)=-1,LSD1=25,LSD2=26,ECUP=53,DRVP=54,XDRP=55,AN1M=56,AN2M=57,AN3M=58,AN4M=59,AN5M=60,AN6M=61,AN7M=62,AN8M=63,AN9M=64,AN10M=65,AN11M=66,AN12M=67,AN13M=68,AN14M=69,AN15M=70,AN16M=71,ESTOP=97,PWMADC=142  altref=5V Reference  typ=uint16  num_adc_bits=12  use_stat=off  use_vardec=off  nam='RTD1_MW'  read_level=1  write_level=1  group='System | I/O Pins | Inputs Config'
  motohawk_ain_read : MotoHawk_lib/Analog I//O Blocks/motohawk_ain_read  nam='PedalSupply'  typ=uint16
  motohawk_probe : MotoHawk_lib/Calibration & Probing Blocks/motohawk_probe  nam='WiperPotRaw'  show_more=off  name_source=Use Parameter  read_level=1  view_as=Number  enum_struct={'Disabled', 'Enabled'}  vector_style=Wide Row  use_help_units=off  help=''  units=''  use_header_enum=off  row_header_enum={}  col_header_enum={}  use_min_max=off  min_val=-inf  max_val=inf  use_precision=off  precision=''  gain=1  offset=0  exp=1  use_mototune_group=off  mototune_group=motohawk_vardec_path(gcb)
  motohawk_probe1 : MotoHawk_lib/Calibration & Probing Blocks/motohawk_probe  nam='WiperPotScaled'  show_more=off  name_source=Use Parameter  read_level=1  view_as=Number  enum_struct={'Disabled', 'Enabled'}  vector_style=Wide Row  use_help_units=off  help=''  units=''  use_header_enum=off  row_header_enum={}  col_header_enum={}  use_min_max=off  min_val=-inf  max_val=inf  use_precision=off  precision=''  gain=1  offset=0  exp=1  use_mototune_group=off  mototune_group=motohawk_vardec_path(gcb)
  motohawk_probe2 : MotoHawk_lib/Calibration & Probing Blocks/motohawk_probe  nam='WiperPotNormalized'  show_more=off  name_source=Use Parameter  read_level=1  view_as=Number  enum_struct={'Disabled', 'Enabled'}  vector_style=Wide Row  use_help_units=off  help=''  units=''  use_header_enum=off  row_header_enum={}  col_header_enum={}  use_min_max=off  min_val=-inf  max_val=inf  use_precision=off  precision=''  gain=1  offset=0  exp=1  use_mototune_group=off  mototune_group=motohawk_vardec_path(gcb)
  motohawk_probe3 : MotoHawk_lib/Calibration & Probing Blocks/motohawk_probe  nam='WiperPot'  show_more=off  name_source=Use Parameter  read_level=1  view_as=Number  enum_struct={'Disabled', 'Enabled'}  vector_style=Wide Row  use_help_units=off  help=''  units=''  use_header_enum=off  row_header_enum={}  col_header_enum={}  use_min_max=off  min_val=-inf  max_val=inf  use_precision=off  precision=''  gain=1  offset=0  exp=1  use_mototune_group=off  mototune_group=motohawk_vardec_path(gcb)
  WiperPot : Outport
  wires:
  motohawk_ain/1 -> Data Type Conversion/1
  motohawk_ain_read/1 -> Data Type Conversion1/1
  Data Type Conversion/1 -> Divide/1, motohawk_probe/1
  Divide/1 -> Gain/1
  Gain/1 -> Wiper Lookup Table/1, motohawk_probe1/1
  Wiper Lookup Table/1 -> Saturation/1, motohawk_probe2/1
  Saturation/1 -> Bus Creator/1, motohawk_probe3/1  "WiperPotPerc"
  Bus Creator/1 -> WiperPot/1
  Data Type Conversion1/1 -> Divide/2

== system GTA_PCMFirmware/Function/1 Inputs and Paramaters/CAN/ Motor Controller ==
  CAN Params : Inport
  Bus Creator : BusCreator
  CurrentFB : Subsystem
  TemperatureWarnFB : Subsystem
  VoltageSpeedFB : Subsystem
  Watchdog : Subsystem
  Kinetek : Outport
  wires:
  CurrentFB/1(KinCurrFdbk) -> Bus Creator/1  "KinCurrFB"
  TemperatureWarnFB/1(KinTempWarn) -> Bus Creator/2  "KinTempWarn"
  VoltageSpeedFB/1(Out1) -> Bus Creator/3  "KinVoltSpeed"
  Watchdog/1(KinWatchdog) -> Bus Creator/4  "KinWatchdog"
  Bus Creator/1 -> Kinetek/1
  CAN Params/1 -> CurrentFB/1(In1), TemperatureWarnFB/1(In1), VoltageSpeedFB/1(In1), Watchdog/1(In1)

== system GTA_PCMFirmware/Function/1 Inputs and Paramaters/CAN/BMS ==
  CAN Params : Inport
  "  Current Sensor" : Subsystem
  " Charger Flags" : Subsystem
  Bus Creator : BusCreator  Inputs=5
  Cell Information : Subsystem
  Cell Temp : Subsystem
  Pack Size : Subsystem
  CurrentSensor : Outport
  wires:
  CAN Params/1 -> "  Current Sensor"/1(CAN Params)
  "  Current Sensor"/1(Current Sensor) -> Bus Creator/1  "csInfo"
  Pack Size/1(PackSize) -> Bus Creator/5  "csPackSize"
  Cell Temp/1(CellTemps) -> Bus Creator/4  "csCellTemps"
  Cell Information/1(Cell Info) -> Bus Creator/3  "csCellInfo"
  " Charger Flags"/1(Charger Flags) -> Bus Creator/2  "csChargeFlags"
  Bus Creator/1 -> CurrentSensor/1
